simulink model "PurePursuit"  (R2021a)
settings: Solver=FixedStepAuto  StartTime=0.0  StopTime=60  FixedStep=0.01  RelTol=1e-3
values from neighbouring files (symbols this model uses):
  kappar = [kr1,kr2,kr3,kr4,kr5,kr6,kr7,kr8,kr9,kr10,kr11]    [routing_planning.m]
  thetar = [theta1,theta2,theta3,theta4,theta5,theta6,theta7,theta8,theta9,theta10,theta11]    [routing_planning.m]
  vr = 6    [routing_planning.m]
  xr = [x1,x2,x3,x4,x5,x6,x7,x8,x9,x10,x11]    [routing_planning.m]
  yr = [y1,y2,y3,y4,y5,y6,y7,y8,y9,y10,y11]    [routing_planning.m]
libraries: autolibshared x1
settings Model: Creator=xiaochangshui  LastModifiedBy=xiaochangshui

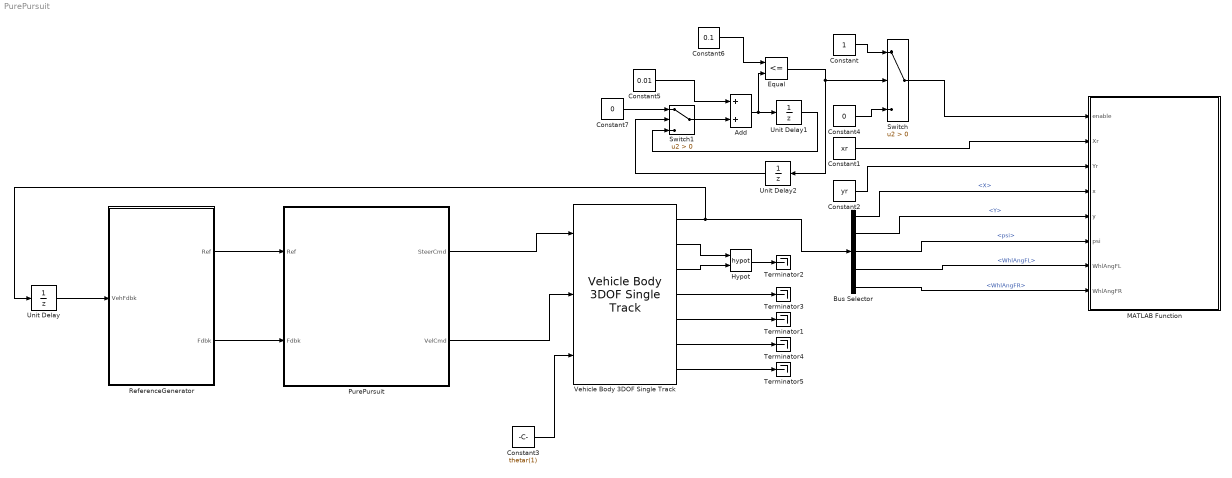
== system PurePursuit ==
  Add : Sum
  Bus Selector : BusSelector  OutputSignals=InertFrm.Cg.Disp.X,InertFrm.Cg.Disp.Y,InertFrm.Cg.Ang.psi,BdyFrm.FrntAxl.Steer.WhlAngFL,BdyFrm.FrntAxl.Steer.WhlAngFR
  Constant : Constant
  Constant1 : Constant  Value=xr  SampleTime=-1
  Constant2 : Constant  Value=yr  SampleTime=-1
  Constant3 : Constant  Value=thetar(1)
  Constant4 : Constant  Value=0
  Constant5 : Constant  Value=0.01
  Constant6 : Constant  Value=0.1
  Constant7 : Constant  Value=0
  Equal : RelationalOperator  Operator=<=  OutDataTypeStr=boolean  RndMeth=Simplest
  Hypot : Math  Operator=hypot  SaturateOnIntegerOverflow=on
  MATLAB Function : MATLAB Function  TreatAsAtomicUnit=on
  PurePursuit : Subsystem  VariantControl=(default)
      mask Display: image('LongitudinalDriver.png'); % Use "Edit Image" on toolstrip to change.
  ReferenceGenerator : Subsystem
  Switch : Switch  Criteria=u2 > Threshold
  Switch1 : Switch  Criteria=u2 > Threshold
  Terminator{1..5} (5 alike) : Terminator
  Unit Delay : UnitDelay  SampleTime=-1  HasFrameUpgradeWarning=on
  Unit Delay1 : UnitDelay  SampleTime=-1  HasFrameUpgradeWarning=on
  Unit Delay2 : UnitDelay  SampleTime=-1  HasFrameUpgradeWarning=on
  Vehicle Body 3DOF Single Track : autolibshared/Vehicle Body 3DOF Single Track  trackMode=Single (bicycle)  inputMode=External longitudinal velocity  frontSteerMode=on  rearSteerMode=off  windMode=off  muMode=off  extFMode=off  extMMode=off  htchFMode=off  htchMMode=off  extXo=off  extpsio=on  extxdoto=off  extro=off  extYo=off  extTamb=off  extydoto=off  aMode=2  NF=2  NR=2  m=2000  a=1.4  b=1.6  h=0.35  dh=1  hh=0.2  X_o=0  xdot_o=0  CalphaMode=off  sigmaMode=on  d=0  hl=0  w=[1.4,1.4]  Cy_f=12e3  Cy_r=11e3  sigma_f=.1  sigma_r=.1  alpha_f_brk=[-.1 .1]  Cy_f_data=[-9e3 9e3]  alpha_r_brk=[-.1 .1]  Cy_r_data=[-9e3 9e3]  Y_o=0  ydot_o=0  Izz=4000  psi_o=0  r_o=0  Af=2  Cd=.3  Cl=.1  Cpm=.1  beta_w=[0:0.01:0.3]  Cs=[0:0.03:0.9]  Cym=[0:0.01:0.3]  Pabs=101325  Tair=273  g=9.81  mu=1  xdot_tol=.01  Fznom=5000  Fxtire_sat=7e4  Fytire_sat=7e4  longOff=0  latOff=0  vertOff=0  wrapAng=off
      settings: SourceProductBaseCode=PW,DR,MT,UV,VE
  wires:
  Vehicle Body 3DOF Single Track/4 -> Terminator3/1
  Vehicle Body 3DOF Single Track/3 -> Hypot/2
  Vehicle Body 3DOF Single Track/1 -> Bus Selector/1, Unit Delay/1
  Vehicle Body 3DOF Single Track/2 -> Hypot/1
  ReferenceGenerator/1(Ref) -> PurePursuit/1(Ref)
  ReferenceGenerator/2(Fdbk) -> PurePursuit/2(Fdbk)
  Hypot/1 -> Terminator2/1
  Vehicle Body 3DOF Single Track/5 -> Terminator1/1
  Vehicle Body 3DOF Single Track/6 -> Terminator4/1
  Vehicle Body 3DOF Single Track/7 -> Terminator5/1
  Unit Delay/1 -> ReferenceGenerator/1(VehFdbk)
  PurePursuit/2(VelCmd) -> Vehicle Body 3DOF Single Track/2
  PurePursuit/1(SteerCmd) -> Vehicle Body 3DOF Single Track/1
  Constant1/1 -> MATLAB Function/2(Xr)
  Constant2/1 -> MATLAB Function/3(Yr)
  Bus Selector/1 -> MATLAB Function/4(x)  "<X>"
  Bus Selector/2 -> MATLAB Function/5(y)  "<Y>"
  Bus Selector/3 -> MATLAB Function/6(psi)  "<psi>"
  Bus Selector/4 -> MATLAB Function/7(WhlAngFL)  "<WhlAngFL>"
  Bus Selector/5 -> MATLAB Function/8(WhlAngFR)  "<WhlAngFR>"
  Switch/1 -> MATLAB Function/1(enable)
  Constant3/1 -> Vehicle Body 3DOF Single Track/3
  Constant/1 -> Switch/1
  Constant4/1 -> Switch/3
  Equal/1 -> Unit Delay2/1, Switch/2
  Constant5/1 -> Add/1
  Add/1 -> Equal/2, Unit Delay1/1
  Unit Delay1/1 -> Switch1/3
  Switch1/1 -> Add/2
  Constant6/1 -> Equal/1
  Constant7/1 -> Switch1/1
  Unit Delay2/1 -> Switch1/2

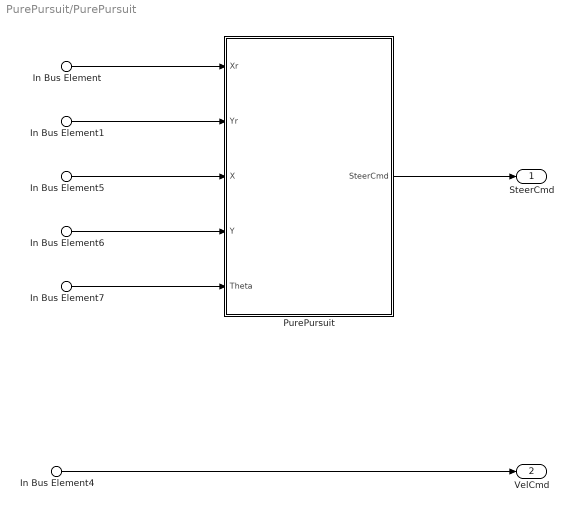
== system PurePursuit/PurePursuit ==
  In Bus Element : Inport  PortName=Ref  Element=X
  In Bus Element1 : Inport  PortName=Ref  Element=Y
  In Bus Element4 : Inport  PortName=Ref  Element=V
  In Bus Element5 : Inport  Port=2  PortName=Fdbk  Element=InertFrm.Cg.Disp.X
  In Bus Element6 : Inport  Port=2  PortName=Fdbk  Element=InertFrm.Cg.Disp.Y
  In Bus Element7 : Inport  Port=2  PortName=Fdbk  Element=InertFrm.Cg.Ang.psi
  PurePursuit : MATLAB Function  TreatAsAtomicUnit=on
  SteerCmd : Outport
  VelCmd : Outport  Port=2
  wires:
  PurePursuit/1(SteerCmd) -> SteerCmd/1
  In Bus Element/1 -> PurePursuit/1(Xr)
  In Bus Element1/1 -> PurePursuit/2(Yr)
  In Bus Element4/1 -> VelCmd/1
  In Bus Element5/1 -> PurePursuit/3(X)
  In Bus Element7/1 -> PurePursuit/5(Theta)
  In Bus Element6/1 -> PurePursuit/4(Y)

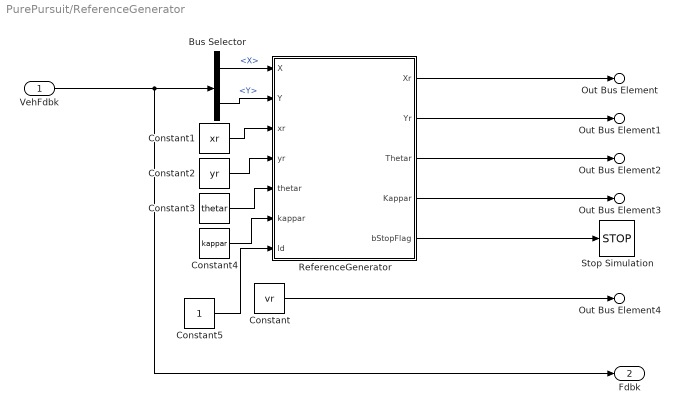
== system PurePursuit/ReferenceGenerator ==
  VehFdbk : Inport
  Bus Selector : BusSelector  OutputSignals=InertFrm.Cg.Disp.X,InertFrm.Cg.Disp.Y
  Constant : Constant  Value=vr  SampleTime=-1
  Constant1 : Constant  Value=xr  SampleTime=-1
  Constant2 : Constant  Value=yr  SampleTime=-1
  Constant3 : Constant  Value=thetar  SampleTime=-1
  Constant4 : Constant  Value=kappar  SampleTime=-1
  Constant5 : Constant
  ReferenceGenerator : MATLAB Function  TreatAsAtomicUnit=on  VariantControl=Choice
  Stop Simulation : Stop
  Out Bus Element : Outport  PortName=Ref  Element=X
  Out Bus Element1 : Outport  PortName=Ref  Element=Y
  Out Bus Element2 : Outport  PortName=Ref  Element=Theta
  Out Bus Element3 : Outport  PortName=Ref  Element=Kappa
  Out Bus Element4 : Outport  PortName=Ref  Element=V
  Fdbk : Outport  Port=2
  wires:
  Bus Selector/1 -> ReferenceGenerator/1(X)  "<X>"
  Bus Selector/2 -> ReferenceGenerator/2(Y)  "<Y>"
  ReferenceGenerator/1(Xr) -> Out Bus Element/1
  ReferenceGenerator/2(Yr) -> Out Bus Element1/1
  ReferenceGenerator/3(Thetar) -> Out Bus Element2/1
  ReferenceGenerator/4(Kappar) -> Out Bus Element3/1
  Constant/1 -> Out Bus Element4/1
  Constant1/1 -> ReferenceGenerator/3(xr)
  Constant2/1 -> ReferenceGenerator/4(yr)
  Constant3/1 -> ReferenceGenerator/5(thetar)
  Constant4/1 -> ReferenceGenerator/6(kappar)
  VehFdbk/1 -> Fdbk/1, Bus Selector/1
  ReferenceGenerator/5(bStopFlag) -> Stop Simulation/1
  Constant5/1 -> ReferenceGenerator/7(ld)

== matlab function PurePursuit/MATLAB Function ==
  data: enable input; Xr input; Yr input; x input; y input; psi input; WhlAngFL input; WhlAngFR input
function fcn(enable, Xr, Yr, x, y, psi, WhlAngFL, WhlAngFR)
    
    if ~enable
        return;
    end
    figure(1)
    clf;
    axis equal;
    hold on;grid on;
    plot(Xr, Yr, 'r', 'LineWidth', 2)
    veh.LB = 2.7;
    veh.LF = 0.95;
    veh.LR = 1.05;
    veh.W = 1.8;
    veh.WR = 0.3;
    xlim(x + [-10, 10])
    ylim(y + [-10, 10])
    
    R = [cos(psi), -sin(psi); sin(psi), cos(psi)]; 
    FL = [x; y] + R * [veh.LB + veh.LF; 0.5 * veh.W];
    FR = [x; y] + R * [veh.LB + veh.LF; -0.5 * veh.W];
    RL = [x; y] + R * [-veh.LR; 0.5 * veh.W];
    RR = [x; y] + R * [-veh.LR; -0.5 * veh.W];
    
    vehx = [FL(1),FR(1),RR(1),RL(1),FL(1)];
    vehy = [FL(2),FR(2),RR(2),RL(2),FL(2)];
    plot(vehx, vehy, 'b', 'LineWidth', 0.5);
    
    FAC = [x; y] + R * [veh.LB; 0.0];
    plot([x, FAC(1)], [y, FAC(2)], 'k', 'LineWidth', 3)
    
    RAL = [x; y] + R * [0.0; 0.5 * veh.W - 0.2];
    RAR = [x; y] + R * [0.0; -0.5 * veh.W + 0.2];
    plot([RAL(1), RAR(1)], [RAL(2), RAR(2)], 'k', 'LineWidth', 3)
    
    FAL = [x; y] + R * [veh.LB; 0.5 * veh.W - 0.2];
    FAR = [x; y] + R * [veh.LB; -0.5 * veh.W + 0.2];
    plot([FAL(1), FAR(1)], [FAL(2), FAR(2)], 'k', 'LineWidth', 3)
    
    RWL1 = [x; y] + R * [veh.WR; 0.5 * veh.W - 0.2];
    RWL2 = [x; y] + R * [-veh.WR; 0.5 * veh.W - 0.2];
    plot([RWL1(1), RWL2(1)], [RWL1(2), RWL2(2)], 'k', 'LineWidth', 3)
    
    RWR1 = [x; y] + R * [veh.WR; -0.5 * veh.W + 0.2];
    RWR2 = [x; y] + R * [-veh.WR; -0.5 * veh.W + 0.2];
    plot([RWR1(1), RWR2(1)], [RWR1(2), RWR2(2)], 'k', 'LineWidth', 3)
    
    FWL1 = [x; y] + R * ([veh.LB; 0.5 * veh.W - 0.2] + veh.WR * [cos(WhlAngFL); sin(WhlAngFL)]);
    FWL2 = [x; y] + R * ([veh.LB; 0.5 * veh.W - 0.2] - veh.WR * [cos(WhlAngFL); sin(WhlAngFL)]);
    plot([FWL1(1), FWL2(1)], [FWL1(2), FWL2(2)], 'k', 'LineWidth', 3)
    
    FWR1 = [x; y] + R * ([veh.LB; -0.5 * veh.W + 0.2] + veh.WR * [cos(WhlAngFR); sin(WhlAngFR)]);
    FWR2 = [x; y] + R * ([veh.LB; -0.5 * veh.W + 0.2] - veh.WR * [cos(WhlAngFR); sin(WhlAngFR)]);
    plot([FWR1(1), FWR2(1)], [FWR1(2), FWR2(2)], 'k', 'LineWidth', 3)
    
    plot(x, y, 'cp') 
end

== matlab function PurePursuit/PurePursuit ==
  data: Xr input; Yr input; X input; Y input; Theta input; SteerCmd output
function SteerCmd  = PurePursuit(Xr, Yr, X, Y, Theta)
    
    ld = sqrt((X - Xr) ^ 2 + (Y - Yr) ^ 2);
    L = 2.7;
    
    ed = (Yr - Y) * cos(Theta) - (Xr - X) * sin(Theta);
    SteerCmd = atan(2.0 * L * ed / ld ^ 2);
    SteerCmd = sign(SteerCmd) * min(1.25*pi /13, abs(SteerCmd));
end

== matlab function PurePursuit/ReferenceGenerator/ReferenceGenerator ==
  settings: updateMethod=DISCRETE
  data: Xr output; X input; Y input; Yr output; Thetar output; Kappar output; xr input; yr input; thetar input; kappar input; bStopFlag output; ld input
function [Xr, Yr, Thetar, Kappar, bStopFlag] = ReferenceGenerator(X, Y, xr, yr, thetar, kappar, ld)

    persistent start_index
    if isempty(start_index)
        start_index = uint32(1);
    end

    for idx = start_index : length(xr)
        if distance(X, Y, xr(idx), yr(idx)) > ld
            start_index = idx;
            break;
        end
    end
    if distance(X, Y, xr(end), yr(end)) < 0.1 && start_index > 0.5 * length(xr)
        bStopFlag = true;
    else
        bStopFlag = false;
    end
    Xr = xr(start_index);
    Yr = yr(start_index);
    Thetar = thetar(start_index);
    Kappar = kappar(start_index);
end

function dist = distance(x1, y1, x2, y2)
   dist = sqrt((x2 - x1) ^ 2 + (y2 - y1) ^ 2); 
end
